simulink model "proyecto_c_fc3"  (R2023b)
settings: Solver=VariableStepAuto  StartTime=0.0  StopTime=0.1  RelTol=1e-3
values from neighbouring files (symbols this model uses):
  test_ts = 9.09090909091e-07    [workspace_proyecto_simulink.mat]
undefined symbols (not defined in the file or in its folder): fdesignblkfcn, gcbh, salida_sintonizador_fc3
(part 1 of 2)
settings Model: Creator=RomaW11  LastModifiedBy=RomaW11

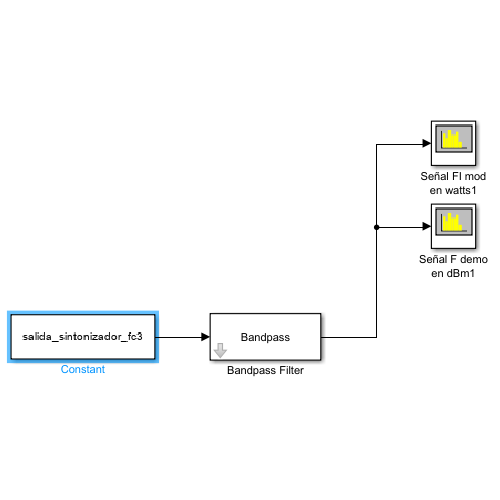
[thumbnail: Simulink's stored preview of the top-level diagram]
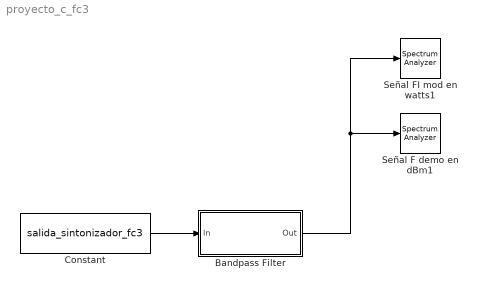
== system proyecto_c_fc3 ==
  Bandpass Filter : Subsystem  DialogController=fdesignblkfcn  InitFcn=fdesignblkfcn(gcbh, {'InitFcn'});  mask(Bandpass Filter){}
      mask help: dsp:DSPFilterDesignBlockDialog:BandpassFdesign_MaskDesc
      settings: CopyFcn=fdesignblkfcn(gcbh, {'CopyFcn'});
      mask Help: helpview(mapfilelocation('dsp'), 'dspbandpassfilter');
      mask Display: disp('Bandpass');
  Constant : Constant  Value=salida_sintonizador_fc3  SampleTime=test_ts
  Señal F demo en dBm1 : SpectrumAnalyzer  WindowPosition=[1.000000,1.000000,1920.000000,1057.000000,]  ScopeFrameLocation=window  SampleRate=44.1e3  StartFrequency=20  StopFrequency=20e3  YLimits=[-108.62580061,38.40656003]  ShowLegend=on  SelectedToolstripTab=spectrumAnalyzerToolstrip.spectrumTab
      settings: OpenAtSimulationStart=off
  Señal FI mod en watts1 : SpectrumAnalyzer  WindowPosition=[1.000000,1.000000,1920.000000,1057.000000,]  ScopeFrameLocation=window  SampleRate=44.1e3  StartFrequency=20  StopFrequency=20e3  SpectrumUnits=Watts  YLimits=[-0.0293253,0.26392767]  ShowLegend=on  SelectedToolstripTab=spectrumAnalyzerToolstrip.spectrumTab
      settings: OpenAtSimulationStart=off
  wires:
  Constant/1 -> Bandpass Filter/1(In)
  Bandpass Filter/1(Out) -> Señal FI mod en watts1/1, Señal F demo en dBm1/1
